simulink model "DrivePattern_harness_model"  (R2022a)
settings: Solver=VariableStepAuto  StartTime=0.0  StopTime=t_end  RelTol=1e-3  AbsTol=1e-3
PreLoadFcn:
  | DrivePattern_harness_setup
libraries: simulink x7
settings Model: Creator=ihctr  LastModifiedBy=isaacito
settings SolverCC: AutoScaleAbsTol=off  AlgebraicLoopSolver=TrustRegion
settings DataIOCC: DSMLogging=off
settings DebuggingCC: UnconnectedInputMsg=warning  UnconnectedOutputMsg=warning  UnconnectedLineMsg=warning  SFMachineParentedDataDiag=warning
settings RTWCC: DLArmComputeVersion=19.05

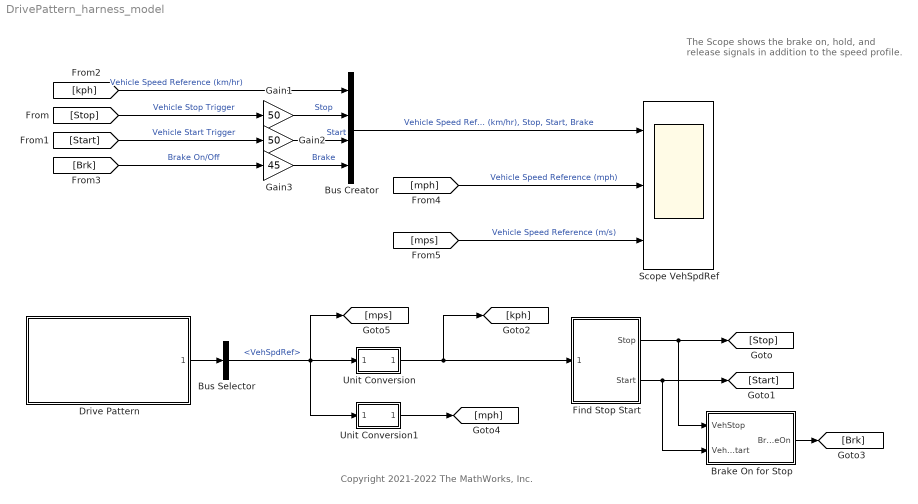
== system DrivePattern_harness_model ==
  note: The Scope shows the brake on,
      | hold, and release signals
      | in addition to the speed profile.
  note: Copyright 2021-2022 The MathWorks, Inc.
  Brake On for Stop : Stateflow chart  TreatAsAtomicUnit=on
  Bus Creator : BusCreator  Inputs=4
  Bus Selector : BusSelector  OutputSignals=VehSpdRef
  Drive Pattern : Subsystem  ReferencedSubsystem=DrivePattern_refsub
  Find Stop Start : Subsystem
  Gain1 : Gain  Gain=50  OutDataTypeStr=double
  Gain2 : Gain  Gain=50  OutDataTypeStr=double
  Gain3 : Gain  Gain=45  OutDataTypeStr=double
  Scope VehSpdRef : Scope  NumInputPorts=3
  Unit Conversion : Subsystem
  Unit Conversion1 : Subsystem
  wires:
  [Stop] -> Gain1/1  "Vehicle Stop Trigger"
  [Start] -> Gain2/1  "Vehicle Start Trigger"
  [Brk] -> Gain3/1  "Brake On/Off"
  Drive Pattern/1 -> Bus Selector/1
  Brake On for Stop/1(BrakeOn) -> [Brk]
  Find Stop Start/2(Start) -> [Start], Brake On for Stop/2(VehStart)
  Find Stop Start/1(Stop) -> [Stop], Brake On for Stop/1(VehStop)
  Bus Selector/1 -> Unit Conversion1/1(In1), Unit Conversion/1(In1), [mps]  "<VehSpdRef>"
  Unit Conversion/1(Out1) -> [kph], Find Stop Start/1(VehSpd)
  Unit Conversion1/1(Out1) -> [mph]
  [kph] -> Bus Creator/1  "Vehicle Speed Reference (km/hr)"
  Gain1/1 -> Bus Creator/2  "Stop"
  Gain2/1 -> Bus Creator/3  "Start"
  Gain3/1 -> Bus Creator/4  "Brake"
  Bus Creator/1 -> Scope VehSpdRef/1  "Vehicle Speed Reference (km/hr), Stop, Start, Brake"
  [mph] -> Scope VehSpdRef/2  "Vehicle Speed Reference (mph)"
  [mps] -> Scope VehSpdRef/3  "Vehicle Speed Reference (m/s)"

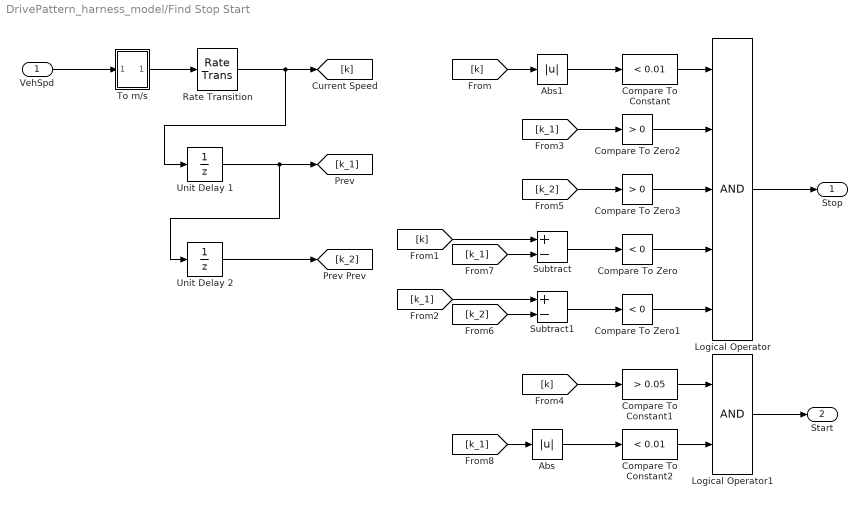
== system DrivePattern_harness_model/Find Stop Start ==
  VehSpd : Inport  Unit=km/hr
  Abs : Abs  SaturateOnIntegerOverflow=off
  Abs1 : Abs  SaturateOnIntegerOverflow=off
  Compare To Constant : simulink/Logic and Bit Operations/Compare To Constant  relop=<  const=0.01  OutDataTypeStr=boolean
  Compare To Constant1 : simulink/Logic and Bit Operations/Compare To Constant  relop=>  const=0.05  OutDataTypeStr=boolean
  Compare To Constant2 : simulink/Logic and Bit Operations/Compare To Constant  relop=<  const=0.01  OutDataTypeStr=boolean
  Compare To Zero : simulink/Logic and Bit Operations/Compare To Zero  relop=<  OutDataTypeStr=boolean
  Compare To Zero1 : simulink/Logic and Bit Operations/Compare To Zero  relop=<  OutDataTypeStr=boolean
  Compare To Zero2 : simulink/Logic and Bit Operations/Compare To Zero  relop=>  OutDataTypeStr=boolean
  Compare To Zero3 : simulink/Logic and Bit Operations/Compare To Zero  relop=>  OutDataTypeStr=boolean
  Logical Operator : Logic  Inputs=5  AllPortsSameDT=off  OutDataTypeStr=boolean
  Logical Operator1 : Logic  AllPortsSameDT=off  OutDataTypeStr=boolean
  Rate Transition : RateTransition  OutPortSampleTime=1
      settings: AttributesFormatString=Sample Time: %<OutPortSampleTime>
  Subtract : Sum  Inputs=+-
  Subtract1 : Sum  Inputs=+-
  To m/s : Subsystem
  Unit Delay 1 : UnitDelay  HasFrameUpgradeWarning=on
      settings: AttributesFormatString=Sample Time: %<SampleTime>
  Unit Delay 2 : UnitDelay  HasFrameUpgradeWarning=on
      settings: AttributesFormatString=Sample Time: %<SampleTime>
  Stop : Outport  OutDataTypeStr=boolean
  Start : Outport  Port=2  OutDataTypeStr=boolean
  wires:
  Rate Transition/1 -> Unit Delay 1/1, [k]
  Subtract/1 -> Compare To Zero/1
  Subtract1/1 -> Compare To Zero1/1
  Compare To Constant/1 -> Logical Operator/1
  Compare To Zero2/1 -> Logical Operator/2
  Compare To Zero1/1 -> Logical Operator/5
  Logical Operator/1 -> Stop/1
  [k] -> Abs1/1
  [k] -> Subtract/1
  [k_1] -> Subtract1/1
  Unit Delay 1/1 -> Unit Delay 2/1, [k_1]
  [k_1] -> Compare To Zero2/1
  Unit Delay 2/1 -> [k_2]
  [k_2] -> Compare To Zero3/1
  [k_2] -> Subtract1/2
  [k_1] -> Subtract/2
  Compare To Zero3/1 -> Logical Operator/3
  Compare To Zero/1 -> Logical Operator/4
  Compare To Constant1/1 -> Logical Operator1/1
  [k] -> Compare To Constant1/1
  [k_1] -> Abs/1
  Compare To Constant2/1 -> Logical Operator1/2
  Logical Operator1/1 -> Start/1
  Abs/1 -> Compare To Constant2/1
  Abs1/1 -> Compare To Constant/1
  VehSpd/1 -> To m/s/1(In1)
  To m/s/1(Out1) -> Rate Transition/1

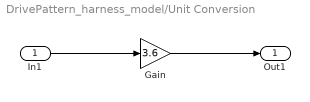
== system DrivePattern_harness_model/Unit Conversion ==
  In1 : Inport  Unit=m/s
  Gain : Gain  Gain=3.6
  Out1 : Outport  OutDataTypeStr=double  Unit=km/hr
  wires:
  Gain/1 -> Out1/1
  In1/1 -> Gain/1

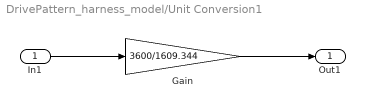
== system DrivePattern_harness_model/Unit Conversion1 ==
  In1 : Inport  Unit=m/s
  Gain : Gain  Gain=3600/1609.344
  Out1 : Outport  OutDataTypeStr=double  Unit=mph
  wires:
  Gain/1 -> Out1/1
  In1/1 -> Gain/1

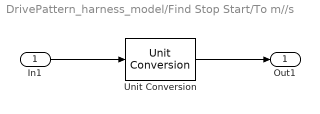
== system DrivePattern_harness_model/Find Stop Start/To m//s ==
  In1 : Inport  Unit=km/hr
  Unit Conversion : UnitConversion
  Out1 : Outport  Unit=m/s
  wires:
  In1/1 -> Unit Conversion/1
  Unit Conversion/1 -> Out1/1

== stateflow chart DrivePattern_harness_model/Brake On for Stop ==
  state BrakeOn
    entry:
    BrakeOn = true;
  state Initial
  state BrakeOff
    entry:
    BrakeOn = false;
  (junction 10) -> BrakeOn : [VehStop == true]
  Initial -> (junction 10) [order 1]
  BrakeOff -> BrakeOn : [VehStop == true]
  BrakeOn -> BrakeOff : [VehStart == true]
  (default) -> Initial
  Initial -> (junction 12) [order 2]
  (junction 12) -> BrakeOff : [VehStart == true]
  data: VehStop input; BrakeOn output; VehStart input
